simulink model "food_control"  (R2018b)
settings: Solver=VariableStepAuto  StartTime=0.0  StopTime=1200  RelTol=1e-3
libraries: simulink x1
settings Model: Creator=esoot  LastModifiedBy=esoot

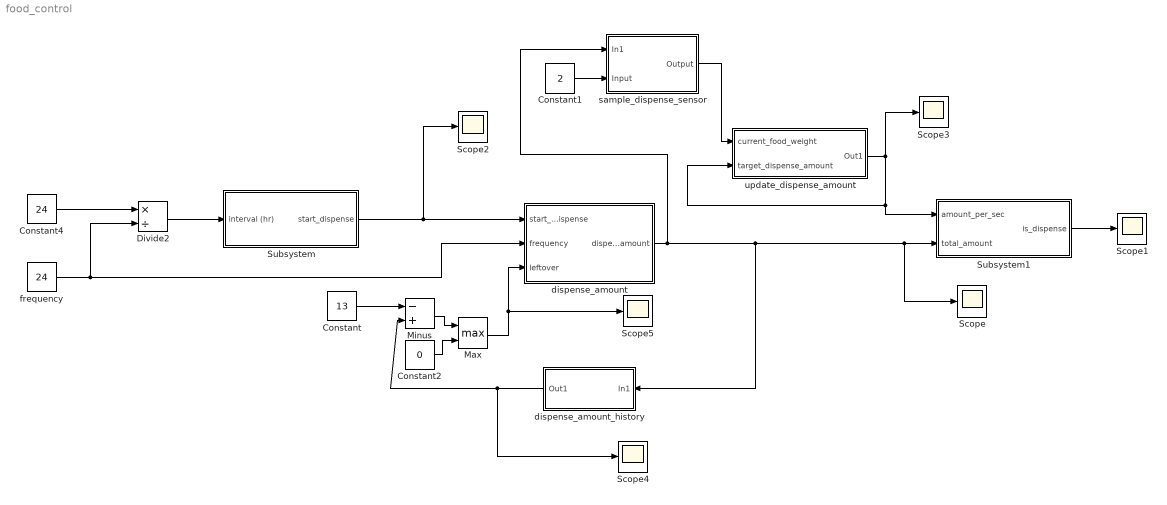
== system food_control ==
  Constant : Constant  Value=13
  Constant1 : Constant  Value=2
  Constant2 : Constant  Value=0
  Constant4 : Constant  Value=24
  Divide2 : Product  Inputs=*/
  Max : MinMax  Function=max  Inputs=2
  Minus : Sum  Inputs=-+
  Scope{,1..5} (6 alike) : Scope
  Subsystem : Subsystem
  Subsystem1 : Subsystem
  dispense_amount : Subsystem
  dispense_amount_history : Subsystem
  frequency : Constant  Value=24
  sample_dispense_sensor : Subsystem
  update_dispense_amount : Subsystem
  wires:
  Divide2/1 -> Subsystem/1(interval (hr))
  Subsystem1/1(is_dispense) -> Scope1/1
  dispense_amount/1(dispense_amount) -> sample_dispense_sensor/1(In1), dispense_amount_history/1(In1), Subsystem1/2(total_amount), Scope/1
  Subsystem/1(start_dispense) -> Scope2/1, dispense_amount/1(start_dispense)
  Constant4/1 -> Divide2/1
  frequency/1 -> Divide2/2, dispense_amount/2(frequency)
  Constant1/1 -> sample_dispense_sensor/2(Input)
  update_dispense_amount/1(Out1) -> Subsystem1/1(amount_per_sec), update_dispense_amount/2(target_dispense_amount), Scope3/1
  sample_dispense_sensor/1(Output) -> update_dispense_amount/1(current_food_weight)
  dispense_amount_history/1(Out1) -> Scope4/1, Minus/2
  Constant/1 -> Minus/1
  Minus/1 -> Max/1
  Constant2/1 -> Max/2
  Max/1 -> dispense_amount/3(leftover), Scope5/1

== system food_control/Subsystem ==
  interval (hr) : Inport
  Constant5 : Constant  Value=0
  Fcn : Fcn  Expr=u*60
  Memory : Memory  InitialCondition=false
  Relational Operator : RelationalOperator  OutDataTypeStr=boolean  RndMeth=Simplest
  interval1 : Subsystem
  start_dispense : Outport
  wires:
  Fcn/1 -> Relational Operator/2
  interval1/1(Output) -> Relational Operator/1
  Relational Operator/1 -> Memory/1, start_dispense/1
  interval (hr)/1 -> Fcn/1
  Memory/1 -> interval1/1(reset)
  Constant5/1 -> interval1/2(init_value)

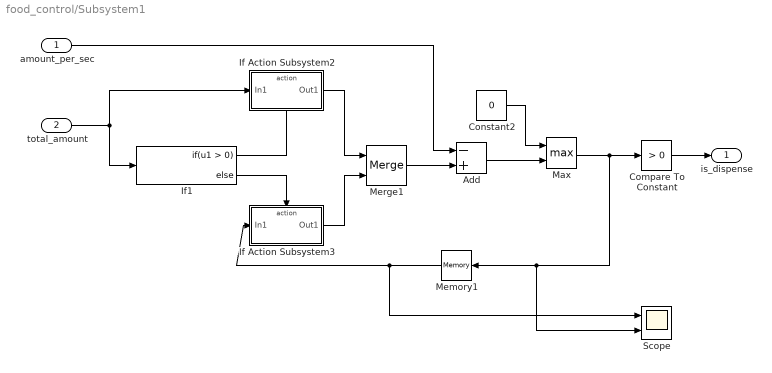
== system food_control/Subsystem1 ==
  amount_per_sec : Inport
  total_amount : Inport  Port=2
  Add : Sum  Inputs=-+
  Compare To Constant : simulink/Logic and Bit Operations/Compare To Constant  relop=>  const=0  OutDataTypeStr=boolean
  Constant2 : Constant  Value=0
  If Action Subsystem2 : Subsystem  TreatAsAtomicUnit=on
  If Action Subsystem3 : Subsystem  TreatAsAtomicUnit=on
  If1 : If
  Max : MinMax  Function=max  Inputs=2
  Memory1 : Memory  LinearizeMemory=on
  Merge1 : Merge
  Scope : Scope  NumInputPorts=2
  is_dispense : Outport
  wires:
  If1/2 -> If Action Subsystem3/Action
  total_amount/1 -> If Action Subsystem2/1(In1), If1/1
  If1/1 -> If Action Subsystem2/Action
  If Action Subsystem3/1(Out1) -> Merge1/2
  If Action Subsystem2/1(Out1) -> Merge1/1
  Add/1 -> Max/2
  Constant2/1 -> Max/1
  amount_per_sec/1 -> Add/1
  Compare To Constant/1 -> is_dispense/1
  Merge1/1 -> Add/2
  Max/1 -> Compare To Constant/1, Memory1/1, Scope/2
  Memory1/1 -> Scope/1, If Action Subsystem3/1(In1)

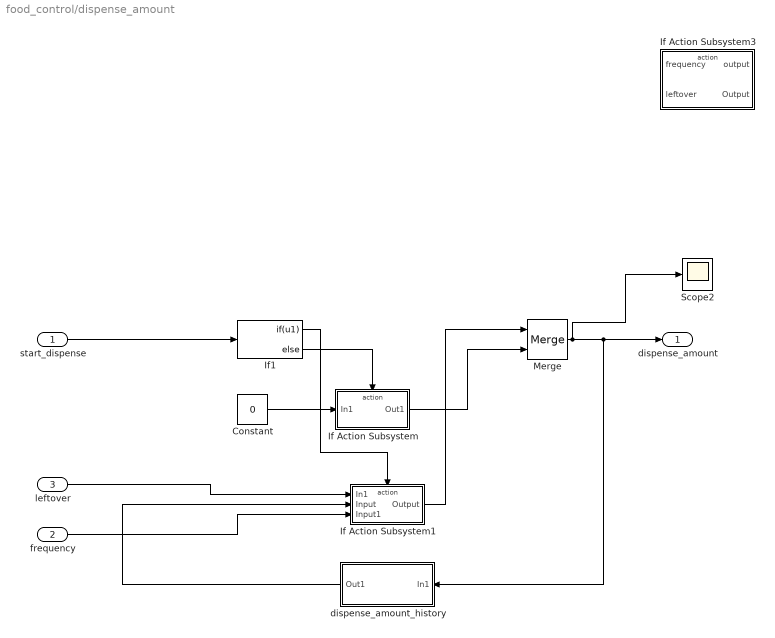
== system food_control/dispense_amount ==
  start_dispense : Inport
  frequency : Inport  Port=2
  leftover : Inport  Port=3
  Constant : Constant  Value=0
  If Action Subsystem : Subsystem  TreatAsAtomicUnit=on
  If Action Subsystem1 : Subsystem  TreatAsAtomicUnit=on
  If Action Subsystem3 : Subsystem  TreatAsAtomicUnit=on
  If1 : If  IfExpression=u1
  Merge : Merge
  Scope2 : Scope
  dispense_amount_history : Subsystem
  dispense_amount : Outport
  wires:
  If1/1 -> If Action Subsystem1/Action
  start_dispense/1 -> If1/1
  leftover/1 -> If Action Subsystem1/1(In1)
  frequency/1 -> If Action Subsystem1/3(Input1)
  If Action Subsystem/1(Out1) -> Merge/2
  If1/2 -> If Action Subsystem/Action
  Constant/1 -> If Action Subsystem/1(In1)
  Merge/1 -> Scope2/1, dispense_amount/1, dispense_amount_history/1(In1)
  dispense_amount_history/1(Out1) -> If Action Subsystem1/2(Input)
  If Action Subsystem1/1(Output) -> Merge/1

== system food_control/dispense_amount_history ==
  In1 : Inport
  If : If  IfExpression=u1 == 0
  If Action Subsystem : Subsystem  TreatAsAtomicUnit=on
  If Action Subsystem1 : Subsystem  TreatAsAtomicUnit=on
  Memory : Memory
  Merge : Merge
  Out1 : Outport
  wires:
  In1/1 -> If Action Subsystem/1(In1), If/1
  If/2 -> If Action Subsystem/Action
  If/1 -> If Action Subsystem1/Action
  Memory/1 -> If Action Subsystem1/1(In1), Out1/1
  If Action Subsystem/1(Out1) -> Merge/2
  If Action Subsystem1/1(Out1) -> Merge/1
  Merge/1 -> Memory/1

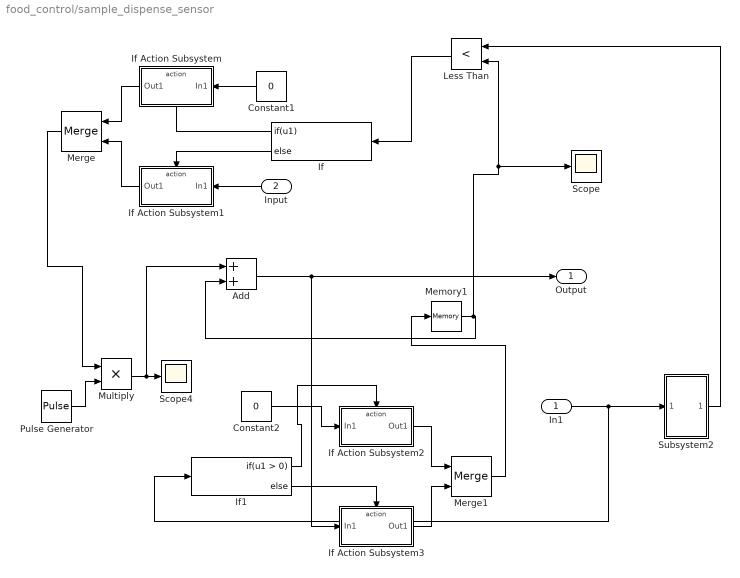
== system food_control/sample_dispense_sensor ==
  In1 : Inport
  Input : Inport  Port=2
  Add : Sum
  Constant1 : Constant  Value=0
  Constant2 : Constant  Value=0
  If : If  IfExpression=u1
  If Action Subsystem : Subsystem  TreatAsAtomicUnit=on
  If Action Subsystem1 : Subsystem  TreatAsAtomicUnit=on
  If Action Subsystem2 : Subsystem  TreatAsAtomicUnit=on
  If Action Subsystem3 : Subsystem  TreatAsAtomicUnit=on
  If1 : If
  Less Than : RelationalOperator  Operator=<  OutDataTypeStr=boolean  RndMeth=Simplest
  Memory1 : Memory
  Merge : Merge
  Merge1 : Merge
  Multiply : Product
  Pulse Generator : DiscretePulseGenerator  PulseType=Time based  Period=1
  Scope : Scope
  Scope4 : Scope
  Subsystem2 : Subsystem
  Output : Outport
  wires:
  In1/1 -> If1/1, Subsystem2/1(In1)
  Add/1 -> Output/1, If Action Subsystem3/1(In1)
  If/1 -> If Action Subsystem/Action
  If/2 -> If Action Subsystem1/Action
  Constant1/1 -> If Action Subsystem/1(In1)
  If Action Subsystem/1(Out1) -> Merge/1
  If Action Subsystem1/1(Out1) -> Merge/2
  Subsystem2/1(Out1) -> Less Than/1
  Less Than/1 -> If/1
  Merge/1 -> Multiply/1
  Input/1 -> If Action Subsystem1/1(In1)
  Pulse Generator/1 -> Multiply/2
  Multiply/1 -> Add/1, Scope4/1
  If1/1 -> If Action Subsystem2/Action
  Constant2/1 -> If Action Subsystem2/1(In1)
  If1/2 -> If Action Subsystem3/Action
  If Action Subsystem2/1(Out1) -> Merge1/1
  If Action Subsystem3/1(Out1) -> Merge1/2
  Merge1/1 -> Memory1/1
  Memory1/1 -> Scope/1, Less Than/2, Add/2

== system food_control/update_dispense_amount ==
  current_food_weight : Inport
  target_dispense_amount : Inport  Port=2
  Scope : Scope
  actual_dispense_amount : Subsystem
  adjust_dispense_amount : Subsystem
  get_error : Subsystem
  Out1 : Outport
  wires:
  actual_dispense_amount/1(Out1) -> get_error/1(actual_dispense_amount)
  adjust_dispense_amount/1(Out1) -> Out1/1, Scope/1
  target_dispense_amount/1 -> adjust_dispense_amount/2(prev_value), get_error/2(target_dispense_amount)
  get_error/1(Out1) -> adjust_dispense_amount/1(error)
  current_food_weight/1 -> actual_dispense_amount/1(In1)

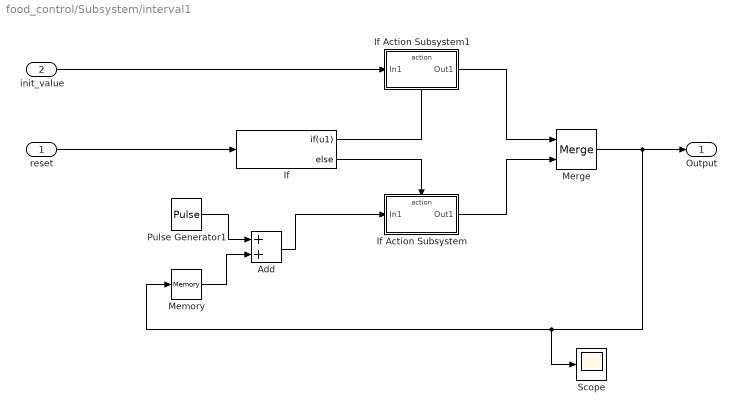
== system food_control/Subsystem/interval1 ==
  reset : Inport
  init_value : Inport  Port=2
  Add : Sum
  If : If  IfExpression=u1
  If Action Subsystem : Subsystem  TreatAsAtomicUnit=on
  If Action Subsystem1 : Subsystem  TreatAsAtomicUnit=on
  Memory : Memory
  Merge : Merge
  Pulse Generator1 : DiscretePulseGenerator  PulseType=Time based  Period=1
  Scope : Scope
  Output : Outport
  wires:
  If/2 -> If Action Subsystem/Action
  If Action Subsystem1/1(Out1) -> Merge/1
  Merge/1 -> Output/1, Scope/1, Memory/1
  init_value/1 -> If Action Subsystem1/1(In1)
  Pulse Generator1/1 -> Add/1
  Add/1 -> If Action Subsystem/1(In1)
  Memory/1 -> Add/2
  If/1 -> If Action Subsystem1/Action
  If Action Subsystem/1(Out1) -> Merge/2
  reset/1 -> If/1

== system food_control/Subsystem1/If Action Subsystem2 ==
  In1 : Inport
  Action Port : ActionPort  ActionType=then
  Out1 : Outport
  wires:
  In1/1 -> Out1/1

== system food_control/Subsystem1/If Action Subsystem3 ==
  In1 : Inport
  Action Port : ActionPort  ActionType=else
  Out1 : Outport
  wires:
  In1/1 -> Out1/1

== system food_control/dispense_amount/If Action Subsystem ==
  In1 : Inport
  Action Port : ActionPort  ActionType=else
  Out1 : Outport
  wires:
  In1/1 -> Out1/1

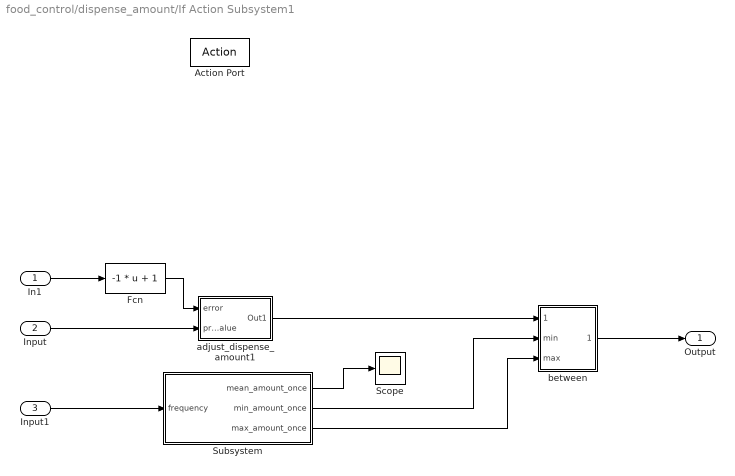
== system food_control/dispense_amount/If Action Subsystem1 ==
  In1 : Inport
  Input : Inport  Port=2
  Input1 : Inport  Port=3
  Action Port : ActionPort  ActionType=then
  Fcn : Fcn  Expr=-1 * u + 1
  Scope : Scope
  Subsystem : Subsystem
  adjust_dispense_amount1 : Subsystem
  between : Subsystem
  Output : Outport
  wires:
  Fcn/1 -> adjust_dispense_amount1/1(error)
  In1/1 -> Fcn/1
  Input/1 -> adjust_dispense_amount1/2(prev_value)
  Subsystem/2(min_amount_once) -> between/2(min)
  Subsystem/3(max_amount_once) -> between/3(max)
  Subsystem/1(mean_amount_once) -> Scope/1
  between/1(Out1) -> Output/1
  adjust_dispense_amount1/1(Out1) -> between/1(value)
  Input1/1 -> Subsystem/1(frequency)

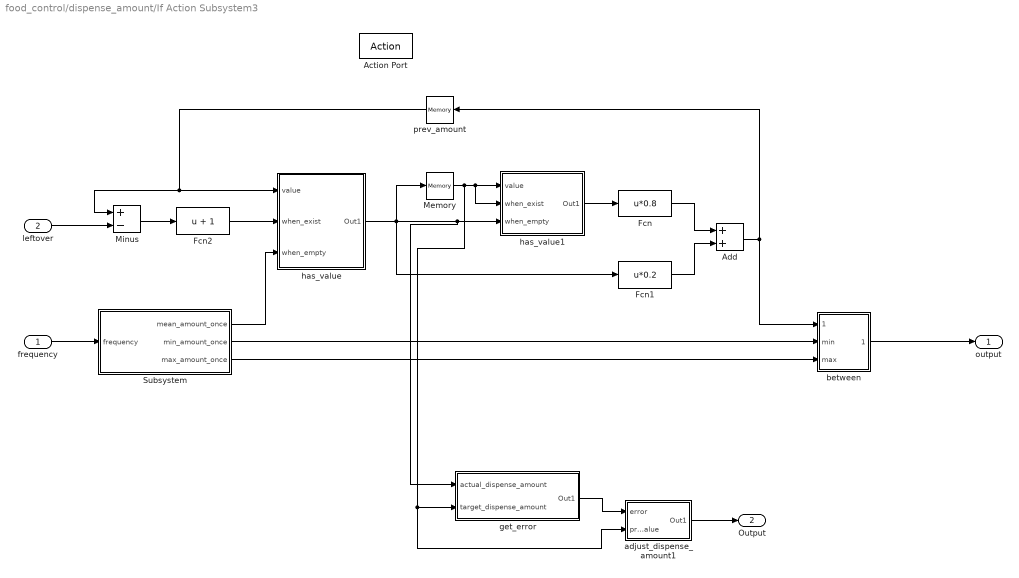
== system food_control/dispense_amount/If Action Subsystem3 ==
  frequency : Inport
  leftover : Inport  Port=2
  Action Port : ActionPort
  Add : Sum
  Fcn : Fcn  Expr=u*0.8
  Fcn1 : Fcn  Expr=u*0.2
  Fcn2 : Fcn  Expr=u + 1
  Memory : Memory
  Minus : Sum  Inputs=+-
  Subsystem : Subsystem
  adjust_dispense_amount1 : Subsystem
  between : Subsystem
  get_error : Subsystem
  has_value : Subsystem
  has_value1 : Subsystem
  prev_amount : Memory  InheritSampleTime=on  LinearizeAsDelay=on
  output : Outport
  Output : Outport  Port=2
  wires:
  Fcn/1 -> Add/1
  has_value/1(Out1) -> Memory/1, Fcn1/1, get_error/1(actual_dispense_amount), has_value1/3(when_empty)
  Minus/1 -> Fcn2/1
  frequency/1 -> Subsystem/1(frequency)
  has_value1/1(Out1) -> Fcn/1
  Fcn1/1 -> Add/2
  prev_amount/1 -> has_value/1(value), Minus/1
  leftover/1 -> Minus/2
  Fcn2/1 -> has_value/2(when_exist)
  Subsystem/1(mean_amount_once) -> has_value/3(when_empty)
  Subsystem/2(min_amount_once) -> between/2(min)
  between/1(Out1) -> output/1
  Add/1 -> prev_amount/1, between/1(value)
  Subsystem/3(max_amount_once) -> between/3(max)
  adjust_dispense_amount1/1(Out1) -> Output/1
  get_error/1(Out1) -> adjust_dispense_amount1/1(error)
  Memory/1 -> adjust_dispense_amount1/2(prev_value), get_error/2(target_dispense_amount), has_value1/2(when_exist), has_value1/1(value)

== system food_control/dispense_amount/dispense_amount_history ==
  In1 : Inport
  If : If  IfExpression=u1 == 0
  If Action Subsystem : Subsystem  TreatAsAtomicUnit=on
  If Action Subsystem1 : Subsystem  TreatAsAtomicUnit=on
  Memory : Memory
  Merge : Merge
  Out1 : Outport
  wires:
  In1/1 -> If Action Subsystem/1(In1), If/1
  If/2 -> If Action Subsystem/Action
  If/1 -> If Action Subsystem1/Action
  Memory/1 -> If Action Subsystem1/1(In1), Out1/1
  If Action Subsystem/1(Out1) -> Merge/2
  If Action Subsystem1/1(Out1) -> Merge/1
  Merge/1 -> Memory/1

== system food_control/dispense_amount_history/If Action Subsystem ==
  In1 : Inport
  Action Port : ActionPort  ActionType=else
  Out1 : Outport
  wires:
  In1/1 -> Out1/1

== system food_control/dispense_amount_history/If Action Subsystem1 ==
  In1 : Inport
  Action Port : ActionPort  ActionType=then
  Out1 : Outport
  wires:
  In1/1 -> Out1/1

== system food_control/sample_dispense_sensor/If Action Subsystem ==
  In1 : Inport
  Action Port : ActionPort  ActionType=then
  Out1 : Outport
  wires:
  In1/1 -> Out1/1

== system food_control/sample_dispense_sensor/If Action Subsystem1 ==
  In1 : Inport
  Action Port : ActionPort  ActionType=else
  Out1 : Outport
  wires:
  In1/1 -> Out1/1

== system food_control/sample_dispense_sensor/If Action Subsystem2 ==
  In1 : Inport
  Action Port : ActionPort  ActionType=then
  Out1 : Outport
  wires:
  In1/1 -> Out1/1

== system food_control/sample_dispense_sensor/If Action Subsystem3 ==
  In1 : Inport
  Action Port : ActionPort  ActionType=else
  Out1 : Outport
  wires:
  In1/1 -> Out1/1

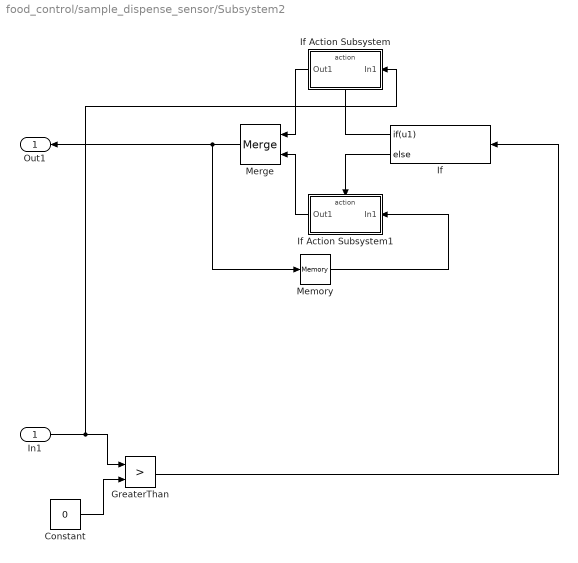
== system food_control/sample_dispense_sensor/Subsystem2 ==
  In1 : Inport
  Constant : Constant  Value=0
  GreaterThan : RelationalOperator  Operator=>  OutDataTypeStr=boolean  RndMeth=Simplest
  If : If  IfExpression=u1
  If Action Subsystem : Subsystem  TreatAsAtomicUnit=on
  If Action Subsystem1 : Subsystem  TreatAsAtomicUnit=on
  Memory : Memory
  Merge : Merge
  Out1 : Outport
  wires:
  In1/1 -> If Action Subsystem/1(In1), GreaterThan/1
  If Action Subsystem/1(Out1) -> Merge/1
  Merge/1 -> Out1/1, Memory/1
  If Action Subsystem1/1(Out1) -> Merge/2
  If/2 -> If Action Subsystem1/Action
  If/1 -> If Action Subsystem/Action
  Memory/1 -> If Action Subsystem1/1(In1)
  Constant/1 -> GreaterThan/2
  GreaterThan/1 -> If/1

== system food_control/update_dispense_amount/actual_dispense_amount ==
  In1 : Inport
  Constant : Constant  Value=0
  Max : MinMax  Function=max  Inputs=2
  Memory : Memory
  Minus : Sum  Inputs=+-
  Out1 : Outport
  wires:
  Constant/1 -> Max/2
  Memory/1 -> Minus/2
  Max/1 -> Out1/1
  Minus/1 -> Max/1
  In1/1 -> Memory/1, Minus/1

== system food_control/update_dispense_amount/adjust_dispense_amount ==
  error : Inport
  prev_value : Inport  Port=2
  Add : Sum
  Fcn : Fcn  Expr=u*0.1
  Memory1 : Memory  InitialCondition=5
  Out1 : Outport
  wires:
  Fcn/1 -> Add/1
  Add/1 -> Memory1/1
  prev_value/1 -> Add/2
  error/1 -> Fcn/1
  Memory1/1 -> Out1/1

== system food_control/update_dispense_amount/get_error ==
  actual_dispense_amount : Inport
  target_dispense_amount : Inport  Port=2
  Minus1 : Sum  Inputs=+-
  if_dispensing : Subsystem
  Out1 : Outport
  wires:
  Minus1/1 -> Out1/1
  if_dispensing/1(Out1) -> Minus1/1
  target_dispense_amount/1 -> Minus1/2, if_dispensing/2(In2)
  actual_dispense_amount/1 -> if_dispensing/1(In1)

== system food_control/Subsystem/interval1/If Action Subsystem ==
  In1 : Inport
  Action Port : ActionPort  ActionType=else
  Out1 : Outport
  wires:
  In1/1 -> Out1/1

== system food_control/Subsystem/interval1/If Action Subsystem1 ==
  In1 : Inport
  Action Port : ActionPort  ActionType=then
  Out1 : Outport
  wires:
  In1/1 -> Out1/1

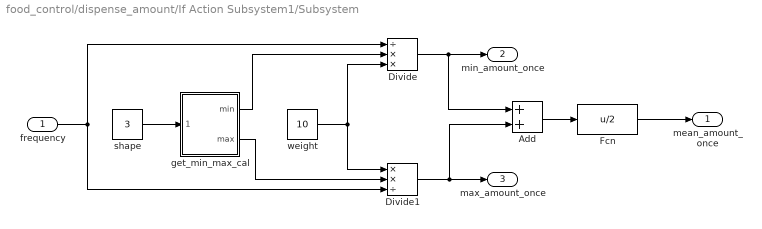
== system food_control/dispense_amount/If Action Subsystem1/Subsystem ==
  frequency : Inport
  Add : Sum
  Divide : Product  Inputs=/**
  Divide1 : Product  Inputs=**/
  Fcn : Fcn  Expr=u/2
  get_min_max_cal : Subsystem
  shape : Constant  Value=3
  weight : Constant  Value=10
  mean_amount_once : Outport
  min_amount_once : Outport  Port=2
  max_amount_once : Outport  Port=3
  wires:
  get_min_max_cal/1(min) -> Divide/2
  frequency/1 -> Divide/1, Divide1/3
  get_min_max_cal/2(max) -> Divide1/2
  weight/1 -> Divide1/1, Divide/3
  shape/1 -> get_min_max_cal/1(shape)
  Add/1 -> Fcn/1
  Divide1/1 -> Add/2, max_amount_once/1
  Divide/1 -> Add/1, min_amount_once/1
  Fcn/1 -> mean_amount_once/1

== system food_control/dispense_amount/If Action Subsystem1/adjust_dispense_amount1 ==
  error : Inport
  prev_value : Inport  Port=2
  Add : Sum
  Fcn : Fcn  Expr=u*0.1
  Memory1 : Memory  InitialCondition=15
  Out1 : Outport
  wires:
  Fcn/1 -> Add/1
  Add/1 -> Memory1/1
  prev_value/1 -> Add/2
  error/1 -> Fcn/1
  Memory1/1 -> Out1/1

== system food_control/dispense_amount/If Action Subsystem1/between ==
  value : Inport
  min : Inport  Port=2
  max : Inport  Port=3
  Max : MinMax  Function=max  Inputs=2
  Max1 : MinMax  Inputs=2
  Out1 : Outport
  wires:
  Max1/1 -> Max/2
  max/1 -> Max1/1
  Max/1 -> Out1/1
  min/1 -> Max/1
  value/1 -> Max1/2

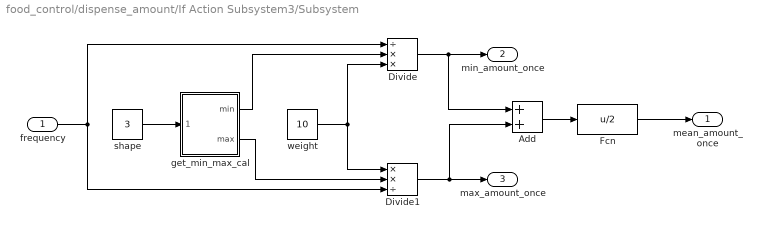
== system food_control/dispense_amount/If Action Subsystem3/Subsystem ==
  frequency : Inport
  Add : Sum
  Divide : Product  Inputs=/**
  Divide1 : Product  Inputs=**/
  Fcn : Fcn  Expr=u/2
  get_min_max_cal : Subsystem
  shape : Constant  Value=3
  weight : Constant  Value=10
  mean_amount_once : Outport
  min_amount_once : Outport  Port=2
  max_amount_once : Outport  Port=3
  wires:
  get_min_max_cal/1(min) -> Divide/2
  frequency/1 -> Divide/1, Divide1/3
  get_min_max_cal/2(max) -> Divide1/2
  weight/1 -> Divide1/1, Divide/3
  shape/1 -> get_min_max_cal/1(shape)
  Add/1 -> Fcn/1
  Divide1/1 -> Add/2, max_amount_once/1
  Divide/1 -> Add/1, min_amount_once/1
  Fcn/1 -> mean_amount_once/1

== system food_control/dispense_amount/If Action Subsystem3/adjust_dispense_amount1 ==
  error : Inport
  prev_value : Inport  Port=2
  Add : Sum
  Fcn : Fcn  Expr=u*0.1
  Memory1 : Memory  InitialCondition=10
  Out1 : Outport
  wires:
  Fcn/1 -> Add/1
  Add/1 -> Memory1/1
  prev_value/1 -> Add/2
  error/1 -> Fcn/1
  Memory1/1 -> Out1/1

== system food_control/dispense_amount/If Action Subsystem3/between ==
  value : Inport
  min : Inport  Port=2
  max : Inport  Port=3
  Max : MinMax  Function=max  Inputs=2
  Max1 : MinMax  Inputs=2
  Out1 : Outport
  wires:
  Max1/1 -> Max/2
  max/1 -> Max1/1
  Max/1 -> Out1/1
  min/1 -> Max/1
  value/1 -> Max1/2

== system food_control/dispense_amount/If Action Subsystem3/get_error ==
  actual_dispense_amount : Inport
  target_dispense_amount : Inport  Port=2
  Minus1 : Sum  Inputs=+-
  if_dispensing : Subsystem
  Out1 : Outport
  wires:
  Minus1/1 -> Out1/1
  if_dispensing/1(Out1) -> Minus1/1
  target_dispense_amount/1 -> Minus1/2, if_dispensing/2(In2)
  actual_dispense_amount/1 -> if_dispensing/1(In1)

== system food_control/dispense_amount/If Action Subsystem3/has_value ==
  value : Inport
  when_exist : Inport  Port=2
  when_empty : Inport  Port=3
  If : If
  If Action Subsystem : Subsystem  TreatAsAtomicUnit=on
  If Action Subsystem1 : Subsystem  TreatAsAtomicUnit=on
  Merge : Merge
  Out1 : Outport
  wires:
  If Action Subsystem1/1(Out1) -> Merge/1
  If/2 -> If Action Subsystem/Action
  If/1 -> If Action Subsystem1/Action
  value/1 -> If/1
  If Action Subsystem/1(Out1) -> Merge/2
  when_empty/1 -> If Action Subsystem/1(In1)
  when_exist/1 -> If Action Subsystem1/1(In1)
  Merge/1 -> Out1/1

== system food_control/dispense_amount/If Action Subsystem3/has_value1 ==
  value : Inport
  when_exist : Inport  Port=2
  when_empty : Inport  Port=3
  If : If
  If Action Subsystem : Subsystem  TreatAsAtomicUnit=on
  If Action Subsystem1 : Subsystem  TreatAsAtomicUnit=on
  Merge : Merge
  Out1 : Outport
  wires:
  If Action Subsystem1/1(Out1) -> Merge/1
  If/2 -> If Action Subsystem/Action
  If/1 -> If Action Subsystem1/Action
  value/1 -> If/1
  If Action Subsystem/1(Out1) -> Merge/2
  when_empty/1 -> If Action Subsystem/1(In1)
  when_exist/1 -> If Action Subsystem1/1(In1)
  Merge/1 -> Out1/1

== system food_control/dispense_amount/dispense_amount_history/If Action Subsystem ==
  In1 : Inport
  Action Port : ActionPort  ActionType=else
  Out1 : Outport
  wires:
  In1/1 -> Out1/1

== system food_control/dispense_amount/dispense_amount_history/If Action Subsystem1 ==
  In1 : Inport
  Action Port : ActionPort  ActionType=then
  Out1 : Outport
  wires:
  In1/1 -> Out1/1

== system food_control/sample_dispense_sensor/Subsystem2/If Action Subsystem ==
  In1 : Inport
  Action Port : ActionPort  ActionType=then
  Out1 : Outport
  wires:
  In1/1 -> Out1/1

== system food_control/sample_dispense_sensor/Subsystem2/If Action Subsystem1 ==
  In1 : Inport
  Action Port : ActionPort  ActionType=else
  Out1 : Outport
  wires:
  In1/1 -> Out1/1

== system food_control/update_dispense_amount/get_error/if_dispensing ==
  In1 : Inport
  In2 : Inport  Port=2
  If : If  IfExpression=u1 == 0
  If Action Subsystem : Subsystem  TreatAsAtomicUnit=on
  If Action Subsystem1 : Subsystem  TreatAsAtomicUnit=on
  Merge : Merge
  Out1 : Outport
  wires:
  If/2 -> If Action Subsystem/Action
  In1/1 -> If/1, If Action Subsystem/1(In1)
  If Action Subsystem1/1(Out1) -> Merge/1
  Merge/1 -> Out1/1
  If/1 -> If Action Subsystem1/Action
  In2/1 -> If Action Subsystem1/1(In1)
  If Action Subsystem/1(Out1) -> Merge/2

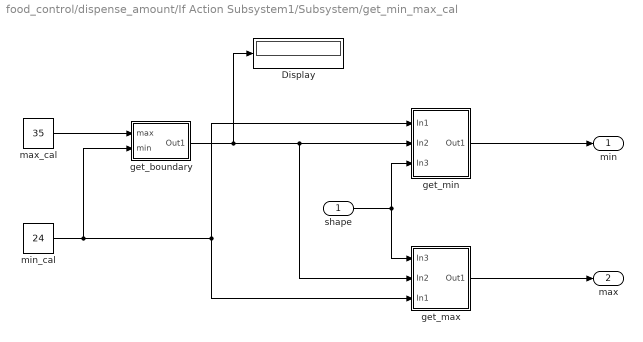
== system food_control/dispense_amount/If Action Subsystem1/Subsystem/get_min_max_cal ==
  shape : Inport
  Display : Display
  get_boundary : Subsystem
  get_max : Subsystem
  get_min : Subsystem
  max_cal : Constant  Value=35
  min_cal : Constant  Value=24
  min : Outport
  max : Outport  Port=2
  wires:
  min_cal/1 -> get_boundary/2(min), get_min/1(In1), get_max/3(In1)
  get_max/1(Out1) -> max/1
  max_cal/1 -> get_boundary/1(max)
  get_boundary/1(Out1) -> Display/1, get_max/2(In2), get_min/2(In2)
  shape/1 -> get_max/1(In3), get_min/3(In3)
  get_min/1(Out1) -> min/1

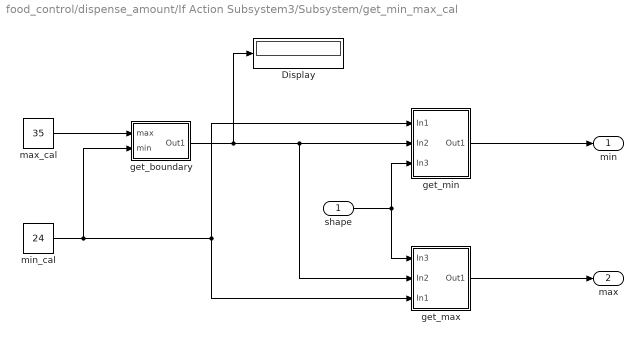
== system food_control/dispense_amount/If Action Subsystem3/Subsystem/get_min_max_cal ==
  shape : Inport
  Display : Display
  get_boundary : Subsystem
  get_max : Subsystem
  get_min : Subsystem
  max_cal : Constant  Value=35
  min_cal : Constant  Value=24
  min : Outport
  max : Outport  Port=2
  wires:
  min_cal/1 -> get_boundary/2(min), get_min/1(In1), get_max/3(In1)
  get_max/1(Out1) -> max/1
  max_cal/1 -> get_boundary/1(max)
  get_boundary/1(Out1) -> Display/1, get_max/2(In2), get_min/2(In2)
  shape/1 -> get_max/1(In3), get_min/3(In3)
  get_min/1(Out1) -> min/1

== system food_control/dispense_amount/If Action Subsystem3/get_error/if_dispensing ==
  In1 : Inport
  In2 : Inport  Port=2
  If : If  IfExpression=u1 == 0
  If Action Subsystem : Subsystem  TreatAsAtomicUnit=on
  If Action Subsystem1 : Subsystem  TreatAsAtomicUnit=on
  Merge : Merge
  Out1 : Outport
  wires:
  If/2 -> If Action Subsystem/Action
  In1/1 -> If/1, If Action Subsystem/1(In1)
  If Action Subsystem1/1(Out1) -> Merge/1
  Merge/1 -> Out1/1
  If/1 -> If Action Subsystem1/Action
  In2/1 -> If Action Subsystem1/1(In1)
  If Action Subsystem/1(Out1) -> Merge/2

== system food_control/dispense_amount/If Action Subsystem3/has_value/If Action Subsystem ==
  In1 : Inport
  Action Port : ActionPort  ActionType=else
  Out1 : Outport
  wires:
  In1/1 -> Out1/1

== system food_control/dispense_amount/If Action Subsystem3/has_value/If Action Subsystem1 ==
  In1 : Inport
  Action Port : ActionPort  ActionType=then
  Out1 : Outport
  wires:
  In1/1 -> Out1/1

== system food_control/dispense_amount/If Action Subsystem3/has_value1/If Action Subsystem ==
  In1 : Inport
  Action Port : ActionPort  ActionType=else
  Out1 : Outport
  wires:
  In1/1 -> Out1/1

== system food_control/dispense_amount/If Action Subsystem3/has_value1/If Action Subsystem1 ==
  In1 : Inport
  Action Port : ActionPort  ActionType=then
  Out1 : Outport
  wires:
  In1/1 -> Out1/1

== system food_control/update_dispense_amount/get_error/if_dispensing/If Action Subsystem ==
  In1 : Inport
  Action Port : ActionPort  ActionType=else
  Out1 : Outport
  wires:
  In1/1 -> Out1/1

== system food_control/update_dispense_amount/get_error/if_dispensing/If Action Subsystem1 ==
  In1 : Inport
  Action Port : ActionPort  ActionType=then
  Out1 : Outport
  wires:
  In1/1 -> Out1/1

== system food_control/dispense_amount/If Action Subsystem1/Subsystem/get_min_max_cal/get_boundary ==
  max : Inport
  min : Inport  Port=2
  Add : Sum  Inputs=-+
  Fcn : Fcn  Expr=u/3
  Out1 : Outport
  wires:
  Add/1 -> Fcn/1
  Fcn/1 -> Out1/1
  min/1 -> Add/1
  max/1 -> Add/2

== system food_control/dispense_amount/If Action Subsystem1/Subsystem/get_min_max_cal/get_max ==
  In3 : Inport
  In2 : Inport  Port=2
  In1 : Inport  Port=3
  Add2 : Sum
  Multiply : Product
  Out1 : Outport
  wires:
  In2/1 -> Multiply/1
  In3/1 -> Multiply/2
  Multiply/1 -> Add2/2
  In1/1 -> Add2/1
  Add2/1 -> Out1/1

== system food_control/dispense_amount/If Action Subsystem1/Subsystem/get_min_max_cal/get_min ==
  In1 : Inport
  In2 : Inport  Port=2
  In3 : Inport  Port=3
  Add1 : Sum
  Fcn1 : Fcn  Expr=u-1
  Multiply1 : Product
  Out1 : Outport
  wires:
  Fcn1/1 -> Multiply1/2
  In2/1 -> Multiply1/1
  Multiply1/1 -> Add1/2
  In3/1 -> Fcn1/1
  In1/1 -> Add1/1
  Add1/1 -> Out1/1

== system food_control/dispense_amount/If Action Subsystem3/Subsystem/get_min_max_cal/get_boundary ==
  max : Inport
  min : Inport  Port=2
  Add : Sum  Inputs=-+
  Fcn : Fcn  Expr=u/3
  Out1 : Outport
  wires:
  Add/1 -> Fcn/1
  Fcn/1 -> Out1/1
  min/1 -> Add/1
  max/1 -> Add/2

== system food_control/dispense_amount/If Action Subsystem3/Subsystem/get_min_max_cal/get_max ==
  In3 : Inport
  In2 : Inport  Port=2
  In1 : Inport  Port=3
  Add2 : Sum
  Multiply : Product
  Out1 : Outport
  wires:
  In2/1 -> Multiply/1
  In3/1 -> Multiply/2
  Multiply/1 -> Add2/2
  In1/1 -> Add2/1
  Add2/1 -> Out1/1

== system food_control/dispense_amount/If Action Subsystem3/Subsystem/get_min_max_cal/get_min ==
  In1 : Inport
  In2 : Inport  Port=2
  In3 : Inport  Port=3
  Add1 : Sum
  Fcn1 : Fcn  Expr=u-1
  Multiply1 : Product
  Out1 : Outport
  wires:
  Fcn1/1 -> Multiply1/2
  In2/1 -> Multiply1/1
  Multiply1/1 -> Add1/2
  In3/1 -> Fcn1/1
  In1/1 -> Add1/1
  Add1/1 -> Out1/1

== system food_control/dispense_amount/If Action Subsystem3/get_error/if_dispensing/If Action Subsystem ==
  In1 : Inport
  Action Port : ActionPort  ActionType=else
  Out1 : Outport
  wires:
  In1/1 -> Out1/1

== system food_control/dispense_amount/If Action Subsystem3/get_error/if_dispensing/If Action Subsystem1 ==
  In1 : Inport
  Action Port : ActionPort  ActionType=then
  Out1 : Outport
  wires:
  In1/1 -> Out1/1
